simulink model "nextpilot_controller"  (R2024b)
settings: Solver=FixedStepAuto  StartTime=0.0  StopTime=inf  FixedStep=5/1000  RelTol=1e-3
undefined symbols (not defined in the file or in its folder): db, Earth, WGS84
libraries: sharedtransform x1, aerolibtransform2 x1
settings Model: DataDictionary=nextpilot_datadict.sldd  Creator=zhanfuyu  LastModifiedBy=CETCA
settings OptimizationCC: ReuseModelBlockBuffer=off
settings RTWCC: GPUComputeCapability=3.5

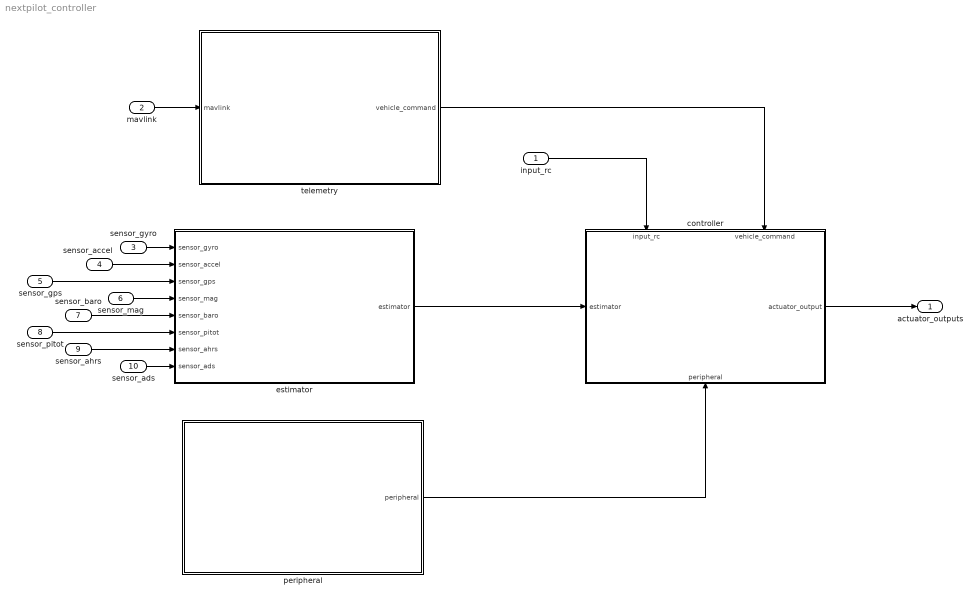
== system nextpilot_controller ==
  input_rc : Inport  OutDataTypeStr=Bus: input_rc_s
  mavlink : Inport  Port=2
  sensor_gyro : Inport  Port=3  OutDataTypeStr=Bus: sensor_gyro_s
  sensor_accel : Inport  Port=4  OutDataTypeStr=Bus: sensor_accel_s
  sensor_gps : Inport  Port=5  OutDataTypeStr=Bus: sensor_gps_s
  sensor_mag : Inport  Port=6  OutDataTypeStr=Bus: sensor_mag_s
  sensor_baro : Inport  Port=7  OutDataTypeStr=Bus: sensor_baro_s
  sensor_pitot : Inport  Port=8  OutDataTypeStr=Bus: differential_pressure_s
  sensor_ahrs : Inport  Port=9  OutDataTypeStr=Bus: sensor_ahrs_s
  sensor_ads : Inport  Port=10  OutDataTypeStr=Bus: sensor_ads_s
  controller : Subsystem
      settings: PortSchema="{\"entries\":[{\"content\":{\"sides\":[{\"content\":{\"connectorIds\":[\"In1\"]},\"type\":\"ConnectorPlacement.EquallySpacedRectSide\",\"uuid\":\"bf365a7c-3df9-4499-baf0-ac7c3d5a0a14\"},{\"content\":{\"connectorIds\":[\"Out1\"],\"side\":\"RIGHT\"},\"type\":\"ConnectorPlacement.EquallySpacedRectSide\",\"uuid\":\"09800274-c410-4406-8158-73f19ad533fb\"},{\"content\":{\"connectorIds\":[\"In2\",\"In3\"],\"side\":\"TOP\"},\"type\":\"ConnectorPlacement.EquallySpacedRectSide\",\"uuid\":\"5f417270-ee37-4bcc-a65c-2cd8f9f9afa3\"},{\"content\":{\"connectorIds\":[\"In4\"],\"side\":\"BOTTOM\"},\"type\":\"ConnectorPlacement.EquallySpacedRectSide\",\"uuid\":\"391e7c1d-4e1b-445f-b382-58d8ebbd70f9\"}]},\"type\":\"ConnectorPlacement.EquallySpacedConnector\",\"uuid\":\"64fe7bf2-fb04-4305-9425-275f1f6f3f70\"}],\"packageUris\":[\"http://schema.mathworks.com/mf0/Connector/R2020b\"],\"version\":\"1.0\"}"
  estimator : Subsystem
  peripheral : Subsystem
  telemetry : Subsystem
  actuator_outputs : Outport  OutDataTypeStr=Bus: actuator_outputs_s
  wires:
  input_rc/1 -> controller/2(input_rc)
  controller/1(actuator_output) -> actuator_outputs/1
  sensor_gyro/1 -> estimator/1(sensor_gyro)
  sensor_accel/1 -> estimator/2(sensor_accel)
  sensor_gps/1 -> estimator/3(sensor_gps)
  sensor_mag/1 -> estimator/4(sensor_mag)
  sensor_baro/1 -> estimator/5(sensor_baro)
  sensor_pitot/1 -> estimator/6(sensor_pitot)
  sensor_ahrs/1 -> estimator/7(sensor_ahrs)
  sensor_ads/1 -> estimator/8(sensor_ads)
  estimator/1(estimator) -> controller/1(estimator)
  mavlink/1 -> telemetry/1(mavlink)
  peripheral/1(peripheral) -> controller/4(peripheral)
  telemetry/1(vehicle_command) -> controller/3(vehicle_command)

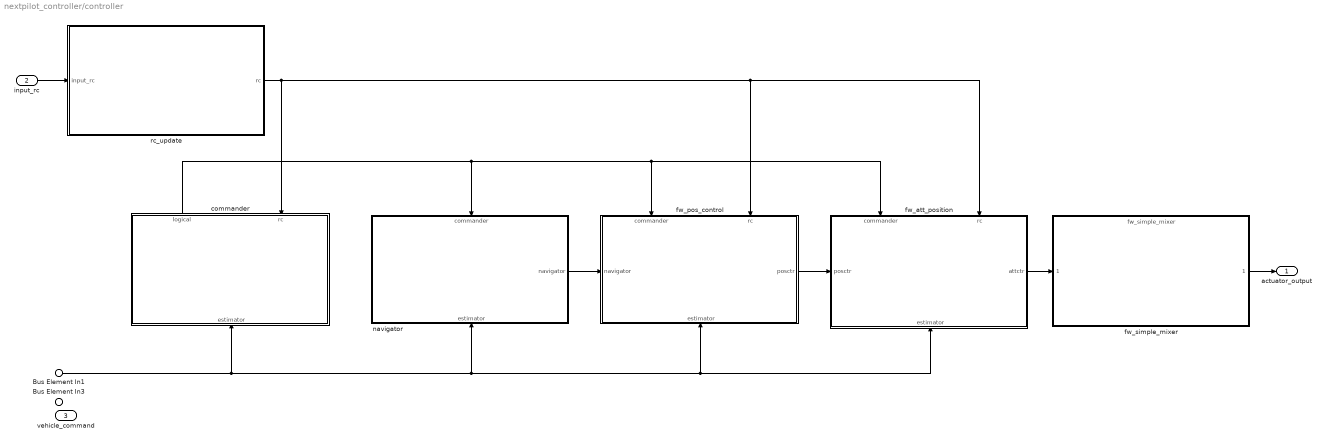
== system nextpilot_controller/controller ==
  Bus Element In1 : Inport  PortName=estimator
  input_rc : Inport  Port=2
  vehicle_command : Inport  Port=3
  Bus Element In3 : Inport  Port=4  PortName=peripheral
  commander : Subsystem
      settings: PortSchema="{\"entries\":[{\"content\":{\"sides\":[{\"content\":{},\"type\":\"ConnectorPlacement.EquallySpacedRectSide\",\"uuid\":\"bf365a7c-3df9-4499-baf0-ac7c3d5a0a14\"},{\"content\":{\"side\":\"RIGHT\"},\"type\":\"ConnectorPlacement.EquallySpacedRectSide\",\"uuid\":\"09800274-c410-4406-8158-73f19ad533fb\"},{\"content\":{\"connectorIds\":[\"Out1\",\"In1\"],\"side\":\"TOP\"},\"type\":\"ConnectorPlacement.EquallySpacedRectSide\",\"uuid\":\"5f417270-ee37-4bcc-a65c-2cd8f9f9afa3\"},{\"content\":{\"connectorIds\":[\"In2\"],\"side\":\"BOTTOM\"},\"type\":\"ConnectorPlacement.EquallySpacedRectSide\",\"uuid\":\"e9383cc9-882d-4d3d-af87-88d70c2eb54b\"}]},\"type\":\"ConnectorPlacement.EquallySpacedConnector\",\"uuid\":\"64fe7bf2-fb04-4305-9425-275f1f6f3f70\"}],\"packageUris\":[\"http://schema.mathworks.com/mf0/Connector/R2020b\"],\"version\":\"1.0\"}"
  fw_att_position : Subsystem
      settings: PortSchema="{\"entries\":[{\"content\":{\"sides\":[{\"content\":{\"connectorIds\":[\"In1\"]},\"type\":\"ConnectorPlacement.EquallySpacedRectSide\",\"uuid\":\"2e5a2222-76bd-46c5-99d4-7bb5e8ecb6d7\"},{\"content\":{\"connectorIds\":[\"Out1\"],\"side\":\"RIGHT\"},\"type\":\"ConnectorPlacement.EquallySpacedRectSide\",\"uuid\":\"0e63d8b1-5138-4700-95dd-60b21314af32\"},{\"content\":{\"connectorIds\":[\"In2\",\"In3\"],\"side\":\"TOP\"},\"type\":\"ConnectorPlacement.EquallySpacedRectSide\",\"uuid\":\"492c5510-7ceb-474c-a2b6-a30ea8da2cdb\"},{\"content\":{\"connectorIds\":[\"In4\"],\"side\":\"BOTTOM\"},\"type\":\"ConnectorPlacement.EquallySpacedRectSide\",\"uuid\":\"7f0239d8-5712-4480-b756-c91313791bd1\"}]},\"type\":\"ConnectorPlacement.EquallySpacedConnector\",\"uuid\":\"77bfd624-d794-4b05-b62c-133b76ce0c6f\"}],\"packageUris\":[\"http://schema.mathworks.com/mf0/Connector/R2020b\"],\"version\":\"1.0\"}"
  fw_pos_control : Subsystem
      settings: PortSchema="{\"entries\":[{\"content\":{\"sides\":[{\"content\":{\"connectorIds\":[\"In1\"]},\"type\":\"ConnectorPlacement.EquallySpacedRectSide\",\"uuid\":\"bf365a7c-3df9-4499-baf0-ac7c3d5a0a14\"},{\"content\":{\"connectorIds\":[\"Out1\"],\"side\":\"RIGHT\"},\"type\":\"ConnectorPlacement.EquallySpacedRectSide\",\"uuid\":\"09800274-c410-4406-8158-73f19ad533fb\"},{\"content\":{\"connectorIds\":[\"In2\",\"In3\"],\"side\":\"TOP\"},\"type\":\"ConnectorPlacement.EquallySpacedRectSide\",\"uuid\":\"5f417270-ee37-4bcc-a65c-2cd8f9f9afa3\"},{\"content\":{\"connectorIds\":[\"In4\"],\"side\":\"BOTTOM\"},\"type\":\"ConnectorPlacement.EquallySpacedRectSide\",\"uuid\":\"f63b4d9c-5df1-47a8-a6da-2d9ff4001925\"}]},\"type\":\"ConnectorPlacement.EquallySpacedConnector\",\"uuid\":\"64fe7bf2-fb04-4305-9425-275f1f6f3f70\"}],\"packageUris\":[\"http://schema.mathworks.com/mf0/Connector/R2020b\"],\"version\":\"1.0\"}"
  fw_simple_mixer : ModelReference  ModelNameDialog=fw_simple_mixer  SimulationMode=Normal  ModelReferenceVersion=1.9
  navigator : Subsystem
      settings: PortSchema="{\"entries\":[{\"content\":{\"sides\":[{\"content\":{},\"type\":\"ConnectorPlacement.EquallySpacedRectSide\",\"uuid\":\"bf365a7c-3df9-4499-baf0-ac7c3d5a0a14\"},{\"content\":{\"connectorIds\":[\"Out1\"],\"side\":\"RIGHT\"},\"type\":\"ConnectorPlacement.EquallySpacedRectSide\",\"uuid\":\"09800274-c410-4406-8158-73f19ad533fb\"},{\"content\":{\"connectorIds\":[\"In1\"],\"side\":\"TOP\"},\"type\":\"ConnectorPlacement.EquallySpacedRectSide\",\"uuid\":\"5f417270-ee37-4bcc-a65c-2cd8f9f9afa3\"},{\"content\":{\"connectorIds\":[\"In2\"],\"side\":\"BOTTOM\"},\"type\":\"ConnectorPlacement.EquallySpacedRectSide\",\"uuid\":\"f0a30678-9212-46d6-bdea-e98ea0374392\"}]},\"type\":\"ConnectorPlacement.EquallySpacedConnector\",\"uuid\":\"64fe7bf2-fb04-4305-9425-275f1f6f3f70\"}],\"packageUris\":[\"http://schema.mathworks.com/mf0/Connector/R2020b\"],\"version\":\"1.0\"}"
  rc_update : Subsystem
  actuator_output : Outport
  wires:
  fw_simple_mixer/1 -> actuator_output/1
  input_rc/1 -> rc_update/1(input_rc)
  commander/1(logical) -> fw_att_position/2(commander), fw_pos_control/2(commander), navigator/1(commander)
  Bus Element In1/1 -> commander/2(estimator), navigator/2(estimator), fw_pos_control/4(estimator), fw_att_position/4(estimator)
  fw_att_position/1(attctr) -> fw_simple_mixer/1
  rc_update/1(rc) -> fw_att_position/3(rc), fw_pos_control/3(rc), commander/1(rc)
  navigator/1(navigator) -> fw_pos_control/1(navigator)
  fw_pos_control/1(posctr) -> fw_att_position/1(posctr)

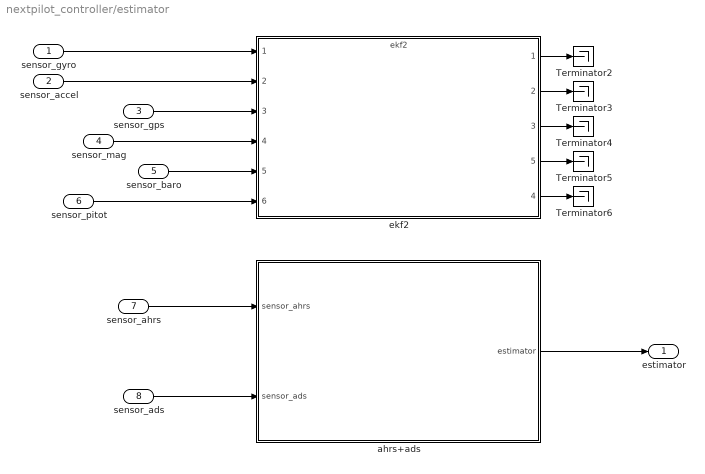
== system nextpilot_controller/estimator ==
  sensor_gyro : Inport
  sensor_accel : Inport  Port=2
  sensor_gps : Inport  Port=3
  sensor_mag : Inport  Port=4
  sensor_baro : Inport  Port=5
  sensor_pitot : Inport  Port=6
  sensor_ahrs : Inport  Port=7
  sensor_ads : Inport  Port=8
  Terminator{2..6} (5 alike) : Terminator
  ahrs+ads : Subsystem
  ekf2 : ModelReference  ModelNameDialog=ekf2.slx  SimulationMode=Normal  ModelReferenceVersion=1.16
      settings: PortSchema="{\"entries\":[{\"content\":{\"sides\":[{\"content\":{\"connectorIds\":[\"In1\",\"In2\",\"In3\",\"In4\",\"In5\",\"In6\"]},\"type\":\"ConnectorPlacement.EquallySpacedRectSide\",\"uuid\":\"530c6754-b0c0-41ce-ae9a-e56605d3448f\"},{\"content\":{\"connectorIds\":[\"Out1\",\"Out2\",\"Out3\",\"Out5\",\"Out4\"],\"side\":\"RIGHT\"},\"type\":\"ConnectorPlacement.EquallySpacedRectSide\",\"uuid\":\"c5c6cdfe-97c8-4b0f-ac33-5a0cc586973e\"},{\"content\":{\"side\":\"TOP\"},\"type\":\"ConnectorPlacement.EquallySpacedRectSide\",\"uuid\":\"89e860c5-fea0-41cc-9e4d-9d1cbdc10ff8\"}]},\"type\":\"ConnectorPlacement.EquallySpacedConnector\",\"uuid\":\"acc5b200-994e-456c-9a09-43fcbf4d1b6b\"}],\"packageUris\":[\"http://schema.mathworks.com/mf0/Connector/R2020b\"],\"version\":\"1.0\"}"
  estimator : Outport
  wires:
  sensor_ahrs/1 -> ahrs+ads/1(sensor_ahrs)
  ekf2/5 -> Terminator5/1
  sensor_gps/1 -> ekf2/3
  ekf2/2 -> Terminator3/1
  ekf2/1 -> Terminator2/1
  ekf2/3 -> Terminator4/1
  sensor_baro/1 -> ekf2/5
  ahrs+ads/1(estimator) -> estimator/1
  sensor_ads/1 -> ahrs+ads/2(sensor_ads)
  ekf2/4 -> Terminator6/1
  sensor_gyro/1 -> ekf2/1
  sensor_accel/1 -> ekf2/2
  sensor_pitot/1 -> ekf2/6
  sensor_mag/1 -> ekf2/4

== system nextpilot_controller/peripheral ==
  Subsystem : Subsystem
  Bus Element Out : Outport  PortName=peripheral  Element=battery_status
  wires:
  Subsystem/1(battery) -> Bus Element Out/1

== system nextpilot_controller/telemetry ==
  mavlink : Inport
  Terminator1 : Terminator
  vehicle_command : Outport
  wires:
  mavlink/1 -> Terminator1/1

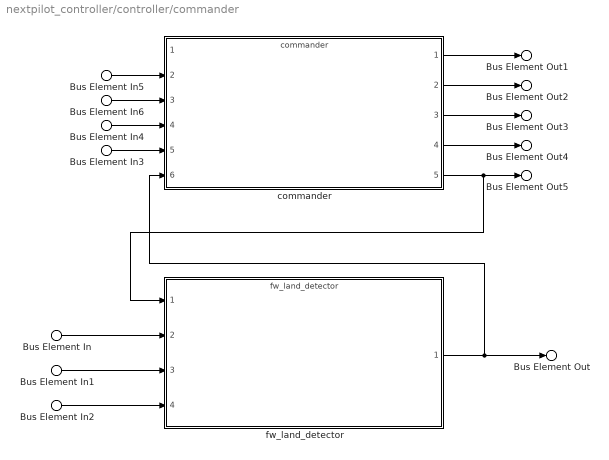
== system nextpilot_controller/controller/commander ==
  Bus Element In5 : Inport  PortName=rc  Element=manual_control_setpoint
  Bus Element In6 : Inport  PortName=rc  Element=manual_control_switches
  Bus Element In1 : Inport  Port=2  PortName=estimator  Element=vehicle_acceleration
  Bus Element In2 : Inport  Port=2  PortName=estimator  Element=airspeed_validated
  Bus Element In4 : Inport  Port=2  PortName=estimator  Element=vehicle_global_position
  Bus Element In : Inport  Port=2  PortName=estimator  Element=vehicle_local_position
  Bus Element In3 : Inport  Port=2  PortName=estimator  Element=vehicle_local_position
  commander : ModelReference  ModelNameDialog=commander  SimulationMode=Normal  ModelReferenceVersion=1.5
  fw_land_detector : ModelReference  ModelNameDialog=fw_land_detector.slx  SimulationMode=Normal  ModelReferenceVersion=1.18
  Bus Element Out : Outport  PortName=logical  Element=vehicle_land_detector
  Bus Element Out1 : Outport  PortName=logical  Element=vehicle_control_mode
  Bus Element Out2 : Outport  PortName=logical  Element=vehicle_status
  Bus Element Out3 : Outport  PortName=logical  Element=vehicle_status_flags
  Bus Element Out4 : Outport  PortName=logical  Element=home_position
  Bus Element Out5 : Outport  PortName=logical  Element=actuator_armed
  wires:
  Bus Element In2/1 -> fw_land_detector/4
  Bus Element In1/1 -> fw_land_detector/3
  Bus Element In/1 -> fw_land_detector/2
  fw_land_detector/1 -> commander/6, Bus Element Out/1
  commander/1 -> Bus Element Out1/1
  commander/2 -> Bus Element Out2/1
  commander/3 -> Bus Element Out3/1
  commander/4 -> Bus Element Out4/1
  commander/5 -> fw_land_detector/1, Bus Element Out5/1
  Bus Element In5/1 -> commander/2
  Bus Element In6/1 -> commander/3
  Bus Element In3/1 -> commander/5
  Bus Element In4/1 -> commander/4

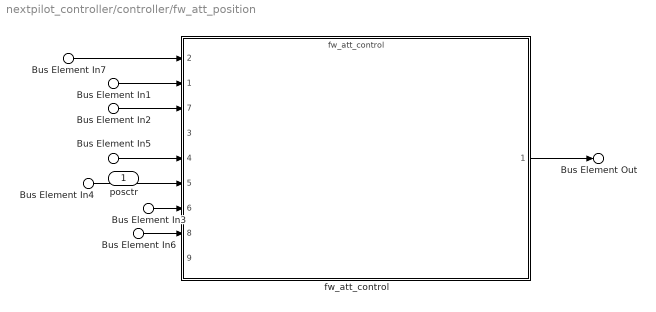
== system nextpilot_controller/controller/fw_att_position ==
  posctr : Inport
  Bus Element In1 : Inport  Port=2  PortName=commander  Element=vehicle_control_mode
  Bus Element In2 : Inport  Port=2  PortName=commander  Element=vehicle_land_detector
  Bus Element In7 : Inport  Port=3  PortName=rc  Element=manual_control_setpoint
  Bus Element In3 : Inport  Port=4  PortName=estimator  Element=airspeed_validated
  Bus Element In6 : Inport  Port=4  PortName=estimator  Element=vehicle_local_position
  Bus Element In4 : Inport  Port=4  PortName=estimator  Element=vehicle_attitude
  Bus Element In5 : Inport  Port=4  PortName=estimator  Element=vehicle_angular_velocity
  fw_att_control : ModelReference  ModelNameDialog=fw_att_control.slx  SimulationMode=Normal  ModelReferenceVersion=1.80
      settings: PortSchema="{\"entries\":[{\"content\":{\"sides\":[{\"content\":{\"connectorIds\":[\"In2\",\"In1\",\"In7\",\"In3\",\"In4\",\"In5\",\"In6\",\"In8\",\"In9\"]},\"type\":\"ConnectorPlacement.EquallySpacedRectSide\",\"uuid\":\"a3897952-0f5d-4f6f-be91-4c088f77e763\"},{\"content\":{\"connectorIds\":[\"Out1\"],\"side\":\"RIGHT\"},\"type\":\"ConnectorPlacement.EquallySpacedRectSide\",\"uuid\":\"30e098fc-1ad2-4a2a-8a05-110c3be1e9a2\"},{\"content\":{\"side\":\"TOP\"},\"type\":\"ConnectorPlacement.EquallySpacedRectSide\",\"uuid\":\"392fb275-10d1-4382-8347-f86adfd12b84\"}]},\"type\":\"ConnectorPlacement.EquallySpacedConnector\",\"uuid\":\"4656b4bb-0794-468e-91b8-e0fd39a991d1\"}],\"packageUris\":[\"http://schema.mathworks.com/mf0/Connector/R2020b\"],\"version\":\"1.0\"}"
  Bus Element Out : Outport  PortName=attctr
  wires:
  Bus Element In4/1 -> fw_att_control/5
  fw_att_control/1 -> Bus Element Out/1
  Bus Element In6/1 -> fw_att_control/8
  Bus Element In3/1 -> fw_att_control/6
  Bus Element In5/1 -> fw_att_control/4
  Bus Element In1/1 -> fw_att_control/1
  Bus Element In2/1 -> fw_att_control/7
  Bus Element In7/1 -> fw_att_control/2

== system nextpilot_controller/controller/fw_pos_control ==
  navigator : Inport
  Bus Element In1 : Inport  Port=2  PortName=commander
  Bus Element In2 : Inport  Port=3  PortName=rc
  Bus Element In3 : Inport  Port=4  PortName=estimator
  posctr : Outport

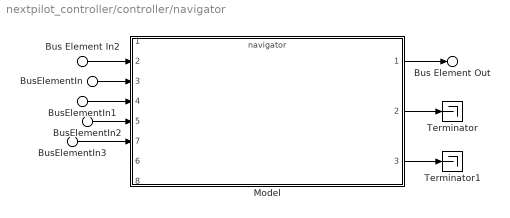
== system nextpilot_controller/controller/navigator ==
  BusElementIn1 : Inport  PortName=commander  Element=vehicle_status
  BusElementIn2 : Inport  PortName=commander  Element=vehicle_land_detector
  BusElementIn3 : Inport  PortName=commander  Element=home_position
  Bus Element In2 : Inport  Port=2  PortName=estimator  Element=vehicle_global_position
  BusElementIn : Inport  Port=2  PortName=estimator  Element=vehicle_local_position
  Model : ModelReference  ModelNameDialog=navigator  SimulationMode=Normal  ModelReferenceVersion=8.108
      settings: PortSchema="{\"entries\":[{\"content\":{\"sides\":[{\"content\":{\"connectorIds\":[\"In1\",\"In2\",\"In3\",\"In4\",\"In5\",\"In7\",\"In6\",\"In8\"]},\"type\":\"ConnectorPlacement.EquallySpacedRectSide\",\"uuid\":\"8fdc0db3-4faf-4964-996f-bada078e6ff8\"},{\"content\":{\"connectorIds\":[\"Out1\",\"Out2\",\"Out3\"],\"side\":\"RIGHT\"},\"type\":\"ConnectorPlacement.EquallySpacedRectSide\",\"uuid\":\"b0bd679b-9745-48c6-a927-6af964e70cab\"},{\"content\":{\"side\":\"TOP\"},\"type\":\"ConnectorPlacement.EquallySpacedRectSide\",\"uuid\":\"ceaa4725-eb95-4176-baf5-413246b64988\"}]},\"type\":\"ConnectorPlacement.EquallySpacedConnector\",\"uuid\":\"98e16fba-50bf-4510-a8fe-8a8b2ebdbf7c\"}],\"packageUris\":[\"http://schema.mathworks.com/mf0/Connector/R2020b\"],\"version\":\"1.0\"}"
  Terminator : Terminator
  Terminator1 : Terminator
  Bus Element Out : Outport  PortName=navigator
  wires:
  Model/2 -> Terminator/1
  Model/3 -> Terminator1/1
  Model/1 -> Bus Element Out/1
  Bus Element In2/1 -> Model/2
  BusElementIn/1 -> Model/3
  BusElementIn2/1 -> Model/5
  BusElementIn1/1 -> Model/4
  BusElementIn3/1 -> Model/7

== system nextpilot_controller/controller/rc_update ==
  input_rc : Inport
  rc_update : ModelReference  ModelNameDialog=rc_update  SimulationMode=Normal  ModelReferenceVersion=8.36
  Bus Element Out : Outport  PortName=rc  Element=manual_control_setpoint
  Bus Element Out1 : Outport  PortName=rc  Element=manual_control_switches
  wires:
  rc_update/1 -> Bus Element Out/1
  rc_update/2 -> Bus Element Out1/1
  input_rc/1 -> rc_update/1

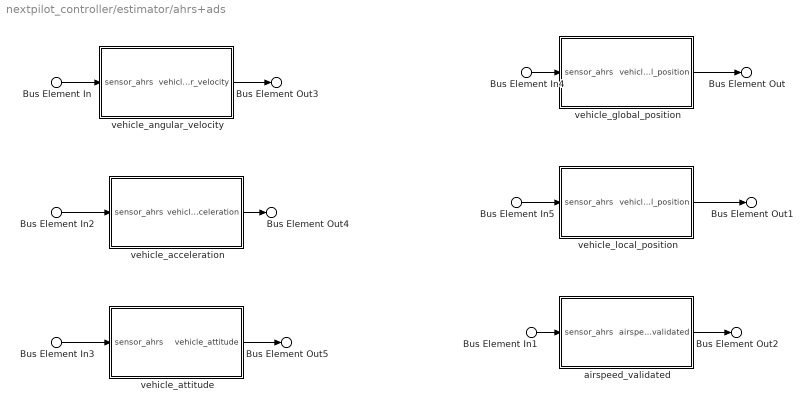
== system nextpilot_controller/estimator/ahrs+ads ==
  Bus Element In{,2..5} (5 alike) : Inport  PortName=sensor_ahrs
  Bus Element In1 : Inport  Port=2  PortName=sensor_ads
  airspeed_validated : Subsystem
  vehicle_acceleration : Subsystem
  vehicle_angular_velocity : Subsystem
  vehicle_attitude : Subsystem
  vehicle_global_position : Subsystem
  vehicle_local_position : Subsystem
  Bus Element Out : Outport  PortName=estimator  Element=vehicle_global_position
  Bus Element Out1 : Outport  PortName=estimator  Element=vehicle_local_position
  Bus Element Out2 : Outport  PortName=estimator  Element=airspeed_validated
  Bus Element Out3 : Outport  PortName=estimator  Element=vehicle_angular_velocity
  Bus Element Out4 : Outport  PortName=estimator  Element=vehicle_acceleration
  Bus Element Out5 : Outport  PortName=estimator  Element=vehicle_attitude
  wires:
  Bus Element In/1 -> vehicle_angular_velocity/1(sensor_ahrs)
  Bus Element In2/1 -> vehicle_acceleration/1(sensor_ahrs)
  Bus Element In3/1 -> vehicle_attitude/1(sensor_ahrs)
  Bus Element In4/1 -> vehicle_global_position/1(sensor_ahrs)
  Bus Element In5/1 -> vehicle_local_position/1(sensor_ahrs)
  Bus Element In1/1 -> airspeed_validated/1(sensor_ahrs)
  vehicle_global_position/1(vehicle_global_position) -> Bus Element Out/1
  vehicle_local_position/1(vehicle_local_position) -> Bus Element Out1/1
  airspeed_validated/1(airspeed_validated) -> Bus Element Out2/1
  vehicle_angular_velocity/1(vehicle_angular_velocity) -> Bus Element Out3/1
  vehicle_acceleration/1(vehicle_acceleration) -> Bus Element Out4/1
  vehicle_attitude/1(vehicle_attitude) -> Bus Element Out5/1

== system nextpilot_controller/peripheral/Subsystem ==
  Constant : Constant  Value=true
  Digital Clock : DigitalClock
  Gain : Gain  Gain=1e6  OutDataTypeStr=uint64
  Bus Element Out : Outport  PortName=battery  Element=timestamp
  Bus Element Out1 : Outport  PortName=battery  Element=connected
  wires:
  Digital Clock/1 -> Gain/1
  Gain/1 -> Bus Element Out/1
  Constant/1 -> Bus Element Out1/1

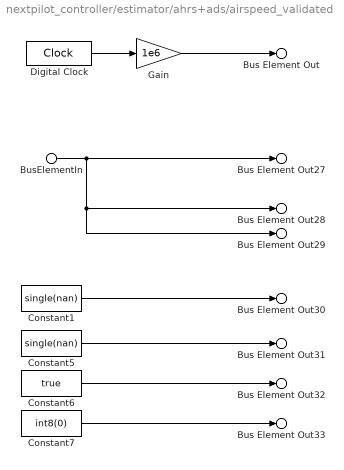
== system nextpilot_controller/estimator/ahrs+ads/airspeed_validated ==
  BusElementIn : Inport  PortName=sensor_ahrs  Element=va
  Constant1 : Constant  Value=single(nan)
  Constant5 : Constant  Value=single(nan)
  Constant6 : Constant  Value=true
  Constant7 : Constant  Value=int8(0)
  Digital Clock : DigitalClock
  Gain : Gain  Gain=1e6  OutDataTypeStr=uint64
  Bus Element Out : Outport  PortName=airspeed_validated  Element=timestamp
  Bus Element Out27 : Outport  PortName=airspeed_validated  Element=indicated_airspeed_m_s
  Bus Element Out28 : Outport  PortName=airspeed_validated  Element=calibrated_airspeed_m_s
  Bus Element Out29 : Outport  PortName=airspeed_validated  Element=true_airspeed_m_s
  Bus Element Out30 : Outport  PortName=airspeed_validated  Element=calibrated_ground_minus_wind_m_s
  Bus Element Out31 : Outport  PortName=airspeed_validated  Element=true_ground_minus_wind_m_s
  Bus Element Out32 : Outport  PortName=airspeed_validated  Element=airspeed_sensor_measurement_valid
  Bus Element Out33 : Outport  PortName=airspeed_validated  Element=selected_airspeed_index
  wires:
  Constant7/1 -> Bus Element Out33/1
  Constant6/1 -> Bus Element Out32/1
  Constant5/1 -> Bus Element Out31/1
  Gain/1 -> Bus Element Out/1
  Digital Clock/1 -> Gain/1
  BusElementIn/1 -> Bus Element Out29/1, Bus Element Out28/1, Bus Element Out27/1
  Constant1/1 -> Bus Element Out30/1

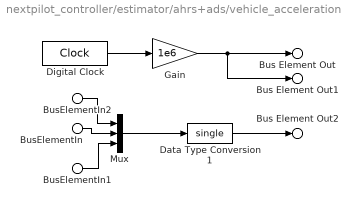
== system nextpilot_controller/estimator/ahrs+ads/vehicle_acceleration ==
  BusElementIn1 : Inport  PortName=sensor_ahrs  Element=az
  BusElementIn : Inport  PortName=sensor_ahrs  Element=ay
  BusElementIn2 : Inport  PortName=sensor_ahrs  Element=ax
  Data Type Conversion1 : DataTypeConversion  OutDataTypeStr=single  SaturateOnIntegerOverflow=off  RndMeth=Floor
  Digital Clock : DigitalClock
  Gain : Gain  Gain=1e6  OutDataTypeStr=uint64
  Mux : Mux  Inputs=3
  Bus Element Out : Outport  PortName=vehicle_acceleration  Element=timestamp
  Bus Element Out1 : Outport  PortName=vehicle_acceleration  Element=timestamp_sample
  Bus Element Out2 : Outport  PortName=vehicle_acceleration  Element=xyz
  wires:
  Data Type Conversion1/1 -> Bus Element Out2/1
  Digital Clock/1 -> Gain/1
  Gain/1 -> Bus Element Out/1, Bus Element Out1/1
  BusElementIn/1 -> Mux/2
  BusElementIn2/1 -> Mux/1
  BusElementIn1/1 -> Mux/3
  Mux/1 -> Data Type Conversion1/1

== system nextpilot_controller/estimator/ahrs+ads/vehicle_angular_velocity ==
  BusElementIn : Inport  PortName=sensor_ahrs  Element=p
  BusElementIn1 : Inport  PortName=sensor_ahrs  Element=q
  BusElementIn2 : Inport  PortName=sensor_ahrs  Element=r
  Digital Clock : DigitalClock
  Gain : Gain  Gain=1e6  OutDataTypeStr=uint64
  Mux : Mux  Inputs=3
  Bus Element Out : Outport  PortName=vehicle_angular_velocity  Element=timestamp
  Bus Element Out1 : Outport  PortName=vehicle_angular_velocity  Element=timestamp_sample
  Bus Element Out2 : Outport  PortName=vehicle_angular_velocity  Element=xyz
  wires:
  Gain/1 -> Bus Element Out1/1, Bus Element Out/1
  Digital Clock/1 -> Gain/1
  BusElementIn1/1 -> Mux/2
  BusElementIn/1 -> Mux/1
  BusElementIn2/1 -> Mux/3
  Mux/1 -> Bus Element Out2/1

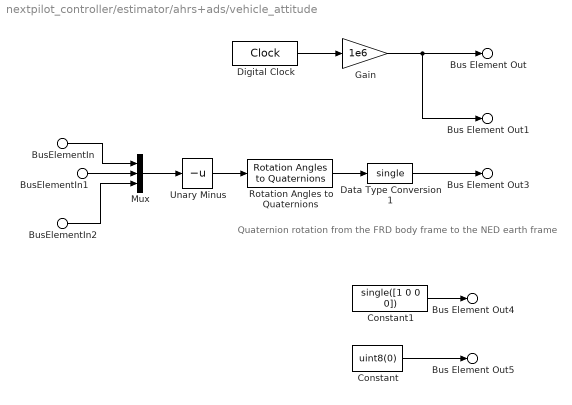
== system nextpilot_controller/estimator/ahrs+ads/vehicle_attitude ==
  note: Quaternion rotation from the FRD body frame to the NED earth frame
  BusElementIn : Inport  PortName=sensor_ahrs  Element=phi
  BusElementIn1 : Inport  PortName=sensor_ahrs  Element=theta
  BusElementIn2 : Inport  PortName=sensor_ahrs  Element=psi
  Constant : Constant  Value=uint8(0)
  Constant1 : Constant  Value=single([1 0 0 0])
  Data Type Conversion1 : DataTypeConversion  OutDataTypeStr=single  SaturateOnIntegerOverflow=off  RndMeth=Floor
  Digital Clock : DigitalClock
  Gain : Gain  Gain=1e6  OutDataTypeStr=uint64
  Mux : Mux  Inputs=3
  Rotation Angles to Quaternions : sharedtransform/Rotation Angles to Quaternions  rotationOrder=XYZ  aMode=aMode
  Unary Minus : UnaryMinus
  Bus Element Out : Outport  PortName=vehicle_attitude  Element=timestamp
  Bus Element Out1 : Outport  PortName=vehicle_attitude  Element=timestamp_sample
  Bus Element Out3 : Outport  PortName=vehicle_attitude  Element=q
  Bus Element Out4 : Outport  PortName=vehicle_attitude  Element=delta_q_reset
  Bus Element Out5 : Outport  PortName=vehicle_attitude  Element=quat_reset_counter
  wires:
  Gain/1 -> Bus Element Out1/1, Bus Element Out/1
  Digital Clock/1 -> Gain/1
  Constant/1 -> Bus Element Out5/1
  Constant1/1 -> Bus Element Out4/1
  Rotation Angles to Quaternions/1 -> Data Type Conversion1/1
  Mux/1 -> Unary Minus/1
  Data Type Conversion1/1 -> Bus Element Out3/1
  Unary Minus/1 -> Rotation Angles to Quaternions/1
  BusElementIn/1 -> Mux/1
  BusElementIn1/1 -> Mux/2
  BusElementIn2/1 -> Mux/3

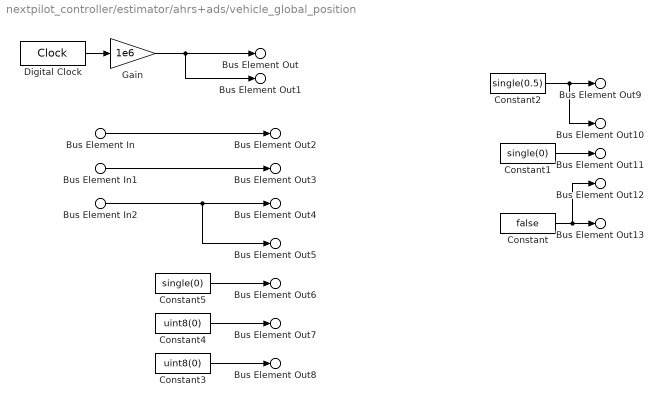
== system nextpilot_controller/estimator/ahrs+ads/vehicle_global_position ==
  Bus Element In : Inport  PortName=sensor_ahrs  Element=lat
  Bus Element In1 : Inport  PortName=sensor_ahrs  Element=lon
  Bus Element In2 : Inport  PortName=sensor_ahrs  Element=alt
  Constant : Constant  Value=false
  Constant1 : Constant  Value=single(0)
  Constant2 : Constant  Value=single(0.5)
  Constant3 : Constant  Value=uint8(0)
  Constant4 : Constant  Value=uint8(0)
  Constant5 : Constant  Value=single(0)
  Digital Clock : DigitalClock
  Gain : Gain  Gain=1e6  OutDataTypeStr=uint64
  Bus Element Out : Outport  PortName=vehicle_global_position  Element=timestamp
  Bus Element Out1 : Outport  PortName=vehicle_global_position  Element=timestamp_sample
  Bus Element Out2 : Outport  PortName=vehicle_global_position  Element=lat
  Bus Element Out3 : Outport  PortName=vehicle_global_position  Element=lon
  Bus Element Out4 : Outport  PortName=vehicle_global_position  Element=alt
  Bus Element Out5 : Outport  PortName=vehicle_global_position  Element=alt_ellipsoid
  Bus Element Out6 : Outport  PortName=vehicle_global_position  Element=delta_alt
  Bus Element Out7 : Outport  PortName=vehicle_global_position  Element=lat_lon_reset_counter
  Bus Element Out8 : Outport  PortName=vehicle_global_position  Element=alt_reset_counter
  Bus Element Out9 : Outport  PortName=vehicle_global_position  Element=eph
  Bus Element Out10 : Outport  PortName=vehicle_global_position  Element=epv
  Bus Element Out11 : Outport  PortName=vehicle_global_position  Element=terrain_alt
  Bus Element Out12 : Outport  PortName=vehicle_global_position  Element=terrain_alt_valid
  Bus Element Out13 : Outport  PortName=vehicle_global_position  Element=dead_reckoning
  wires:
  Constant/1 -> Bus Element Out12/1, Bus Element Out13/1
  Constant1/1 -> Bus Element Out11/1
  Constant2/1 -> Bus Element Out10/1, Bus Element Out9/1
  Constant3/1 -> Bus Element Out8/1
  Constant4/1 -> Bus Element Out7/1
  Constant5/1 -> Bus Element Out6/1
  Digital Clock/1 -> Gain/1
  Gain/1 -> Bus Element Out1/1, Bus Element Out/1
  Bus Element In2/1 -> Bus Element Out5/1, Bus Element Out4/1
  Bus Element In1/1 -> Bus Element Out3/1
  Bus Element In/1 -> Bus Element Out2/1

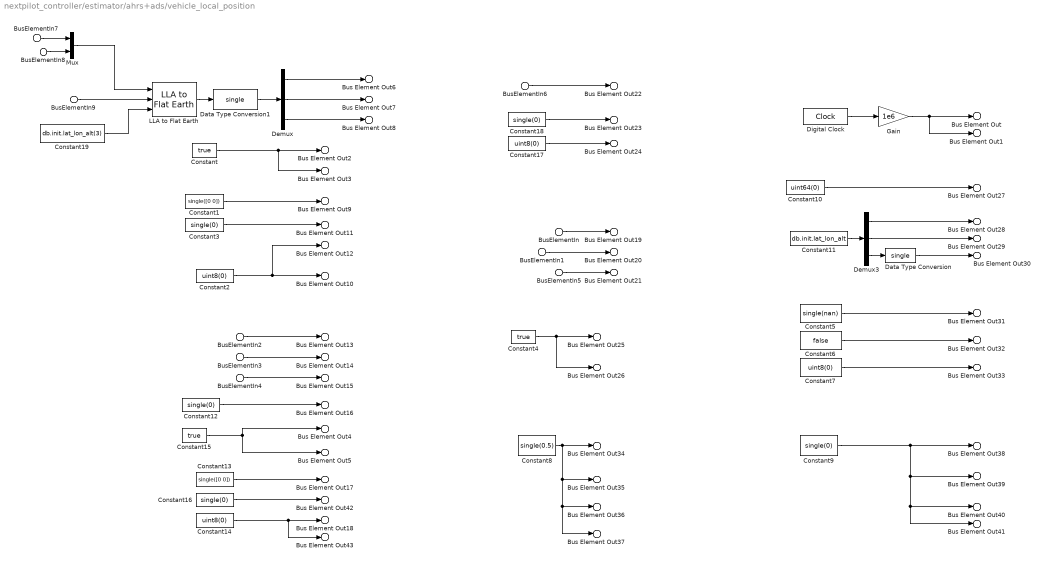
== system nextpilot_controller/estimator/ahrs+ads/vehicle_local_position ==
  BusElementIn2 : Inport  PortName=sensor_ahrs  Element=vn
  BusElementIn3 : Inport  PortName=sensor_ahrs  Element=ve
  BusElementIn4 : Inport  PortName=sensor_ahrs  Element=vd
  BusElementIn : Inport  PortName=sensor_ahrs  Element=ax
  BusElementIn1 : Inport  PortName=sensor_ahrs  Element=ay
  BusElementIn5 : Inport  PortName=sensor_ahrs  Element=az
  BusElementIn6 : Inport  PortName=sensor_ahrs  Element=psi
  BusElementIn7 : Inport  PortName=sensor_ahrs  Element=lat
  BusElementIn8 : Inport  PortName=sensor_ahrs  Element=lon
  BusElementIn9 : Inport  PortName=sensor_ahrs  Element=alt
  Constant : Constant  Value=true
  Constant1 : Constant  Value=single([0 0])
  Constant10 : Constant  Value=uint64(0)
  Constant11 : Constant  Value=db.init.lat_lon_alt
  Constant{3,9,12,16,18} (5 alike) : Constant  Value=single(0)
  Constant13 : Constant  Value=single([0 0])
  Constant{2,7,14,17} (4 alike) : Constant  Value=uint8(0)
  Constant15 : Constant  Value=true
  Constant19 : Constant  Value=db.init.lat_lon_alt(3)
  Constant4 : Constant  Value=true
  Constant5 : Constant  Value=single(nan)
  Constant6 : Constant  Value=false
  Constant8 : Constant  Value=single(0.5)
  Data Type Conversion : DataTypeConversion  OutDataTypeStr=single  SaturateOnIntegerOverflow=off  RndMeth=Floor
  Data Type Conversion1 : DataTypeConversion  OutDataTypeStr=single  SaturateOnIntegerOverflow=off  RndMeth=Floor
  Demux : Demux  Outputs=3
  Demux3 : Demux  Outputs=3
  Digital Clock : DigitalClock
  Gain : Gain  Gain=1e6  OutDataTypeStr=uint64
  LLA to Flat Earth : aerolibtransform2/LLA to Flat Earth  units=Metric (MKS)  ptype=Earth (WGS84)  F=1/298.257223563  R=6378137  refPosPort=off  LL0=db.init.lat_lon_alt(1:2)  psi=0
  Mux : Mux  Inputs=2
  Bus Element Out : Outport  PortName=vehicle_local_position  Element=timestamp
  Bus Element Out1 : Outport  PortName=vehicle_local_position  Element=timestamp_sample
  Bus Element Out2 : Outport  PortName=vehicle_local_position  Element=xy_valid
  Bus Element Out3 : Outport  PortName=vehicle_local_position  Element=z_valid
  Bus Element Out4 : Outport  PortName=vehicle_local_position  Element=v_xy_valid
  Bus Element Out5 : Outport  PortName=vehicle_local_position  Element=v_z_valid
  Bus Element Out6 : Outport  PortName=vehicle_local_position  Element=x
  Bus Element Out7 : Outport  PortName=vehicle_local_position  Element=y
  Bus Element Out8 : Outport  PortName=vehicle_local_position  Element=z
  Bus Element Out9 : Outport  PortName=vehicle_local_position  Element=delta_xy
  Bus Element Out10 : Outport  PortName=vehicle_local_position  Element=xy_reset_counter
  Bus Element Out11 : Outport  PortName=vehicle_local_position  Element=delta_z
  Bus Element Out12 : Outport  PortName=vehicle_local_position  Element=z_reset_counter
  Bus Element Out13 : Outport  PortName=vehicle_local_position  Element=vx
  Bus Element Out14 : Outport  PortName=vehicle_local_position  Element=vy
  Bus Element Out15 : Outport  PortName=vehicle_local_position  Element=vz
  Bus Element Out16 : Outport  PortName=vehicle_local_position  Element=z_deriv
  Bus Element Out17 : Outport  PortName=vehicle_local_position  Element=delta_vxy
  Bus Element Out18 : Outport  PortName=vehicle_local_position  Element=vxy_reset_counter
  Bus Element Out42 : Outport  PortName=vehicle_local_position  Element=delta_vz
  Bus Element Out43 : Outport  PortName=vehicle_local_position  Element=vz_reset_counter
  Bus Element Out19 : Outport  PortName=vehicle_local_position  Element=ax
  Bus Element Out20 : Outport  PortName=vehicle_local_position  Element=ay
  Bus Element Out21 : Outport  PortName=vehicle_local_position  Element=az
  Bus Element Out22 : Outport  PortName=vehicle_local_position  Element=heading
  Bus Element Out23 : Outport  PortName=vehicle_local_position  Element=delta_heading
  Bus Element Out24 : Outport  PortName=vehicle_local_position  Element=heading_reset_counter
  Bus Element Out25 : Outport  PortName=vehicle_local_position  Element=xy_global
  Bus Element Out26 : Outport  PortName=vehicle_local_position  Element=z_global
  Bus Element Out27 : Outport  PortName=vehicle_local_position  Element=ref_timestamp
  Bus Element Out28 : Outport  PortName=vehicle_local_position  Element=ref_lat
  Bus Element Out29 : Outport  PortName=vehicle_local_position  Element=ref_lon
  Bus Element Out30 : Outport  PortName=vehicle_local_position  Element=ref_alt
  Bus Element Out31 : Outport  PortName=vehicle_local_position  Element=dist_bottom
  Bus Element Out32 : Outport  PortName=vehicle_local_position  Element=dist_bottom_valid
  Bus Element Out33 : Outport  PortName=vehicle_local_position  Element=dist_bottom_sensor_bitfield
  Bus Element Out34 : Outport  PortName=vehicle_local_position  Element=eph
  Bus Element Out35 : Outport  PortName=vehicle_local_position  Element=epv
  Bus Element Out36 : Outport  PortName=vehicle_local_position  Element=evh
  Bus Element Out37 : Outport  PortName=vehicle_local_position  Element=evv
  Bus Element Out38 : Outport  PortName=vehicle_local_position  Element=vxy_max
  Bus Element Out39 : Outport  PortName=vehicle_local_position  Element=vz_max
  Bus Element Out40 : Outport  PortName=vehicle_local_position  Element=hagl_min
  Bus Element Out41 : Outport  PortName=vehicle_local_position  Element=hagl_max
  wires:
  Digital Clock/1 -> Gain/1
  Gain/1 -> Bus Element Out1/1, Bus Element Out/1
  Constant/1 -> Bus Element Out3/1, Bus Element Out2/1
  Constant1/1 -> Bus Element Out9/1
  Constant2/1 -> Bus Element Out12/1, Bus Element Out10/1
  Constant3/1 -> Bus Element Out11/1
  Constant4/1 -> Bus Element Out26/1, Bus Element Out25/1
  Constant5/1 -> Bus Element Out31/1
  Constant6/1 -> Bus Element Out32/1
  Constant7/1 -> Bus Element Out33/1
  Constant8/1 -> Bus Element Out37/1, Bus Element Out36/1, Bus Element Out35/1, Bus Element Out34/1
  Constant9/1 -> Bus Element Out39/1, Bus Element Out40/1, Bus Element Out41/1, Bus Element Out38/1
  Demux/2 -> Bus Element Out7/1
  Demux/1 -> Bus Element Out6/1
  Demux/3 -> Bus Element Out8/1
  BusElementIn3/1 -> Bus Element Out14/1
  BusElementIn2/1 -> Bus Element Out13/1
  BusElementIn4/1 -> Bus Element Out15/1
  Constant10/1 -> Bus Element Out27/1
  Constant11/1 -> Demux3/1
  Demux3/3 -> Data Type Conversion/1
  Demux3/2 -> Bus Element Out29/1
  Demux3/1 -> Bus Element Out28/1
  Data Type Conversion/1 -> Bus Element Out30/1
  Constant12/1 -> Bus Element Out16/1
  Constant13/1 -> Bus Element Out17/1
  Constant14/1 -> Bus Element Out43/1, Bus Element Out18/1
  Constant15/1 -> Bus Element Out5/1, Bus Element Out4/1
  Constant16/1 -> Bus Element Out42/1
  Constant17/1 -> Bus Element Out24/1
  Constant18/1 -> Bus Element Out23/1
  BusElementIn6/1 -> Bus Element Out22/1
  BusElementIn/1 -> Bus Element Out19/1
  BusElementIn1/1 -> Bus Element Out20/1
  BusElementIn5/1 -> Bus Element Out21/1
  Constant19/1 -> LLA to Flat Earth/3
  BusElementIn7/1 -> Mux/1
  BusElementIn8/1 -> Mux/2
  Mux/1 -> LLA to Flat Earth/1
  BusElementIn9/1 -> LLA to Flat Earth/2
  LLA to Flat Earth/1 -> Data Type Conversion1/1
  Data Type Conversion1/1 -> Demux/1
